simulink model "PM"  (R2021b)
settings: Solver=VariableStepAuto  StartTime=0.0  StopTime=10  MaxStep=0.00001  RelTol=1e-3
libraries: commanapbnd3 x1
settings Model: Creator=user  LastModifiedBy=USER

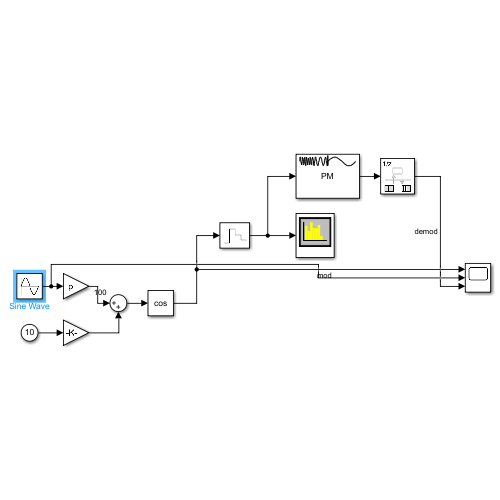
[thumbnail: Simulink's stored preview of the top-level diagram]
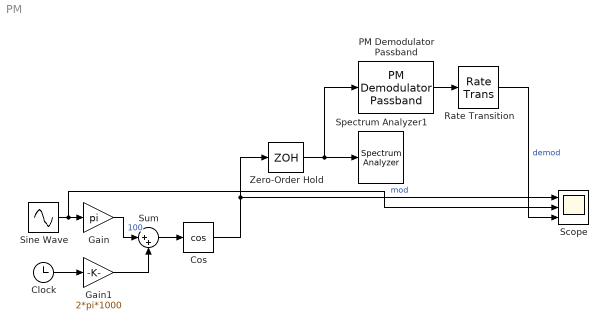
== system PM ==
  Clock : Clock
  Cos : Trigonometry  Operator=cos
  Gain : Gain  Gain=pi
  Gain1 : Gain  Gain=2*pi*1000
  PM Demodulator Passband : commanapbnd3/PM Demodulator Passband  Fc=1000  Ph=0  Kc=pi  Ho=100
      settings: SourceProductBaseCode=CM
  Rate Transition : RateTransition
  Scope : Scope  NumInputPorts=3
  Sine Wave : Sin  Frequency=100 * 2 * pi  SampleTime=0
  Spectrum Analyzer1 : SpectrumAnalyzer
  Sum : Sum  Inputs=|++
  Zero-Order Hold : ZeroOrderHold  SampleTime=1e-4
  wires:
  Sine Wave/1 -> Scope/2, Gain/1
  Clock/1 -> Gain1/1
  Gain1/1 -> Sum/2
  Sum/1 -> Cos/1
  Cos/1 -> Zero-Order Hold/1, Scope/1  "mod"
  Zero-Order Hold/1 -> PM Demodulator Passband/1, Spectrum Analyzer1/1
  Gain/1 -> Sum/1  "100"
  PM Demodulator Passband/1 -> Rate Transition/1
  Rate Transition/1 -> Scope/3  "demod"
